simulink model "SF011A_EotLrng"  (R2013b)
settings: Solver=FixedStepDiscrete  SolverMode=SingleTasking  StartTime=0.0  StopTime=1  FixedStep=0.002  RelTol=1e-3
values from neighbouring files (symbols this model uses):
  ARCHGLBPRM_FLOATZEROTHD_ULS_F32 = DataDict.Constant    [SF011A_EotLrng_DataDict.m]
  CNVTOMILLISEC_MILLISECPERCNT_F32 = DataDict.Constant    [SF011A_EotLrng_DataDict.m]
  CORRLNFLT_CNT_U08 = DataDict.Constant    [SF011A_EotLrng_DataDict.m]
  DEBSTEP_CNT_U16 = DataDict.Constant    [SF011A_EotLrng_DataDict.m]
  EOTLIMDETD_CNT_LOGL = DataDict.Constant    [SF011A_EotLrng_DataDict.m]
  EOTLIMNOTDETD_CNT_LOGL = DataDict.Constant    [SF011A_EotLrng_DataDict.m]
  EotLrngAuthyStrtLrn = DataDict.Calibration    [SF011A_EotLrng_DataDict.m]
  EotLrngEotLrnTmr = DataDict.Calibration    [SF011A_EotLrng_DataDict.m]
  EotLrngHwAgOverTrvlCnt = DataDict.Calibration    [SF011A_EotLrng_DataDict.m]
  EotLrngHwAgOverTrvlEntr = DataDict.Calibration    [SF011A_EotLrng_DataDict.m]
  EotLrngHwAgOverTrvlExit = DataDict.Calibration    [SF011A_EotLrng_DataDict.m]
  EotLrngHwTqEotLrn = DataDict.Calibration    [SF011A_EotLrng_DataDict.m]
  EotLrngMotVelEotLrn = DataDict.Calibration    [SF011A_EotLrng_DataDict.m]
  EotLrngRackTrvlMax = DataDict.Calibration    [SF011A_EotLrng_DataDict.m]
  EotLrngRackTrvlMin = DataDict.Calibration    [SF011A_EotLrng_DataDict.m]
  EotLrngRstAuthyMin = DataDict.Calibration    [SF011A_EotLrng_DataDict.m]
  EotProtnRackTrvlLimrEna = DataDict.ImprtdCal    [SF011A_EotLrng_DataDict.m]
  HwAgOverTrvl = DataDict.NTC    [SF011A_EotLrng_DataDict.m]
  HWAGOVERTRVLMAXCNT_CNT_U08 = DataDict.Constant    [SF011A_EotLrng_DataDict.m]
  NODEBSTEP_CNT_U16 = DataDict.Constant    [SF011A_EotLrng_DataDict.m]
  OUTOFRNGFLT_CNT_U08 = DataDict.Constant    [SF011A_EotLrng_DataDict.m]
  RackEotStorgFlt = DataDict.NTC    [SF011A_EotLrng_DataDict.m]
  SIGAVLFLT_CNT_U08 = DataDict.Constant    [SF011A_EotLrng_DataDict.m]
undefined symbols (not defined in the file or in its folder): NtcSts1, NvmGetErrSts1, SigQlfr1
libraries: simulink x19, NxtrNvM x12, NxtrAbslt x5, NxtrLim x4, NxtrMax x3, NxtrMin x3
(part 7 of 7)

== system SF011A_EotLrng/EotLrng/EotLrngPer1/SRLNotEna/LrnEotLim/LrgnEotCmplSts/EotCwElpdTmr/GetTiSpan100MicroSec32bit/Wrapping/CopyRight2 ==

== stateflow chart SF011A_EotLrng/EotLrng/EotLrngPer1/SRLEna/ChkEotSigForNtc/EotSigAvl/SetCorrlFltNtc/SetNtcSts/ISO Fault Debounce Design ==
  note: NTCSTS_PASSD           (0)
      | NTCSTS_FAILD             (1)
      | NTCSTS_PREPASSD   (2)
      | NTCSTS_PREFAILD     (3)
      |
      | SIGQLFR_NORES        (0)
      | SIGQLFR_PASSD         (1)
      | SIGQLFR_FAILD           (2)
  note: Pass Loop
  note: Fail Loop
  note: 
  (default) -> (junction 89)
  (junction 89) -> (junction 95) [order 1] : [NtcSts ==3]
  (junction 89) -> (junction 93) [order 2] : [NtcSts ==2]
  (junction 89) -> (junction 141) [order 3] : [NtcSts ==1]
      | { ErrAcc = 32767;
      | Qualifier =2;
      |  }
  (junction 89) -> (junction 141) [order 4] : [NtcSts ==0]
      | { ErrAcc = -32768;
      | Qualifier=1;
      | }
  (junction 95) -> (junction 103) [order 2]
  (junction 95) -> (junction 111) [order 1] : [ErrAcc <=0]
      | {ErrAcc = DebStep;}
  (junction 93) -> (junction 123) [order 2] : {
      | ErrAcc = ErrAcc - DebStep;
      | }
  (junction 93) -> (junction 123) [order 1] : [(ErrAcc - DebStep) <= -32768]
      | { ErrAcc = -32768;
      | Qualifier=1;
      | }
  (junction 103) -> (junction 111) [order 1] : [(ErrAcc + DebStep) <32767]
      | {ErrAcc = ErrAcc + DebStep;}
  (junction 103) -> (junction 111) [order 2] : {ErrAcc = 32767;
      | Qualifier =2;}
  (junction 123) -> (junction 141)
  (junction 111) -> (junction 141)
  (junction 141) -> (junction 159) [order 2] : {ErrAcc = 0;
      | Qualifier =0;
      | }
  (junction 141) -> (junction 159) [order 1] : [SvcClr ==0]
  data: NtcSts input Enum: NtcSts1; Qualifier output uint8; DebStep input uint16; ErrAcc local single; SvcClr input

== stateflow chart SF011A_EotLrng/EotLrng/EotLrngPer1/SRLEna/ChkEotSigForNtc/SetSigAvlFltNtc/SetNtcSts/ISO Fault Debounce Design ==
  note: NTCSTS_PASSD           (0)
      | NTCSTS_FAILD             (1)
      | NTCSTS_PREPASSD   (2)
      | NTCSTS_PREFAILD     (3)
      |
      | SIGQLFR_NORES        (0)
      | SIGQLFR_PASSD         (1)
      | SIGQLFR_FAILD           (2)
  note: Pass Loop
  note: Fail Loop
  note: 
  (default) -> (junction 89)
  (junction 89) -> (junction 95) [order 1] : [NtcSts ==3]
  (junction 89) -> (junction 93) [order 2] : [NtcSts ==2]
  (junction 89) -> (junction 141) [order 3] : [NtcSts ==1]
      | { ErrAcc = 32767;
      | Qualifier =2;
      |  }
  (junction 89) -> (junction 141) [order 4] : [NtcSts ==0]
      | { ErrAcc = -32768;
      | Qualifier=1;
      | }
  (junction 95) -> (junction 103) [order 2]
  (junction 95) -> (junction 111) [order 1] : [ErrAcc <=0]
      | {ErrAcc = DebStep;}
  (junction 93) -> (junction 123) [order 2] : {
      | ErrAcc = ErrAcc - DebStep;
      | }
  (junction 93) -> (junction 123) [order 1] : [(ErrAcc - DebStep) <= -32768]
      | { ErrAcc = -32768;
      | Qualifier=1;
      | }
  (junction 103) -> (junction 111) [order 1] : [(ErrAcc + DebStep) <32767]
      | {ErrAcc = ErrAcc + DebStep;}
  (junction 103) -> (junction 111) [order 2] : {ErrAcc = 32767;
      | Qualifier =2;}
  (junction 123) -> (junction 141)
  (junction 111) -> (junction 141)
  (junction 141) -> (junction 159) [order 2] : {ErrAcc = 0;
      | Qualifier =0;
      | }
  (junction 141) -> (junction 159) [order 1] : [SvcClr ==0]
  data: NtcSts input Enum: NtcSts1; Qualifier output uint8; DebStep input uint16; ErrAcc local single; SvcClr input

== stateflow chart SF011A_EotLrng/EotLrng/EotLrngPer1/SRLEna/ChkEotSigForNtc/EotSigAvl/SetOutOfRngNtc/SetNtcSts/ISO Fault Debounce Design ==
  note: NTCSTS_PASSD           (0)
      | NTCSTS_FAILD             (1)
      | NTCSTS_PREPASSD   (2)
      | NTCSTS_PREFAILD     (3)
      |
      | SIGQLFR_NORES        (0)
      | SIGQLFR_PASSD         (1)
      | SIGQLFR_FAILD           (2)
  note: Pass Loop
  note: Fail Loop
  note: 
  (default) -> (junction 89)
  (junction 89) -> (junction 95) [order 1] : [NtcSts ==3]
  (junction 89) -> (junction 93) [order 2] : [NtcSts ==2]
  (junction 89) -> (junction 141) [order 3] : [NtcSts ==1]
      | { ErrAcc = 32767;
      | Qualifier =2;
      |  }
  (junction 89) -> (junction 141) [order 4] : [NtcSts ==0]
      | { ErrAcc = -32768;
      | Qualifier=1;
      | }
  (junction 95) -> (junction 103) [order 2]
  (junction 95) -> (junction 111) [order 1] : [ErrAcc <=0]
      | {ErrAcc = DebStep;}
  (junction 93) -> (junction 123) [order 2] : {
      | ErrAcc = ErrAcc - DebStep;
      | }
  (junction 93) -> (junction 123) [order 1] : [(ErrAcc - DebStep) <= -32768]
      | { ErrAcc = -32768;
      | Qualifier=1;
      | }
  (junction 103) -> (junction 111) [order 1] : [(ErrAcc + DebStep) <32767]
      | {ErrAcc = ErrAcc + DebStep;}
  (junction 103) -> (junction 111) [order 2] : {ErrAcc = 32767;
      | Qualifier =2;}
  (junction 123) -> (junction 141)
  (junction 111) -> (junction 141)
  (junction 141) -> (junction 159) [order 2] : {ErrAcc = 0;
      | Qualifier =0;
      | }
  (junction 141) -> (junction 159) [order 1] : [SvcClr ==0]
  data: NtcSts input Enum: NtcSts1; Qualifier output uint8; DebStep input uint16; ErrAcc local single; SvcClr input

== stateflow chart SF011A_EotLrng/EotLrng/EotLrngPer1/HwAgCwAndCcwMax/HwAgCwAndCcw/OverTrvlDiagc/CntOvrTrvlAndSetNTC/SetOverTrvlDiagc/SetNtcSts/ISO Fault Debounce Design ==
  note: NTCSTS_PASSD           (0)
      | NTCSTS_FAILD             (1)
      | NTCSTS_PREPASSD   (2)
      | NTCSTS_PREFAILD     (3)
      |
      | SIGQLFR_NORES        (0)
      | SIGQLFR_PASSD         (1)
      | SIGQLFR_FAILD           (2)
  note: Pass Loop
  note: Fail Loop
  note: 
  (default) -> (junction 89)
  (junction 89) -> (junction 95) [order 1] : [NtcSts ==3]
  (junction 89) -> (junction 93) [order 2] : [NtcSts ==2]
  (junction 89) -> (junction 141) [order 3] : [NtcSts ==1]
      | { ErrAcc = 32767;
      | Qualifier =2;
      |  }
  (junction 89) -> (junction 141) [order 4] : [NtcSts ==0]
      | { ErrAcc = -32768;
      | Qualifier=1;
      | }
  (junction 95) -> (junction 103) [order 2]
  (junction 95) -> (junction 111) [order 1] : [ErrAcc <=0]
      | {ErrAcc = DebStep;}
  (junction 93) -> (junction 123) [order 2] : {
      | ErrAcc = ErrAcc - DebStep;
      | }
  (junction 93) -> (junction 123) [order 1] : [(ErrAcc - DebStep) <= -32768]
      | { ErrAcc = -32768;
      | Qualifier=1;
      | }
  (junction 103) -> (junction 111) [order 1] : [(ErrAcc + DebStep) <32767]
      | {ErrAcc = ErrAcc + DebStep;}
  (junction 103) -> (junction 111) [order 2] : {ErrAcc = 32767;
      | Qualifier =2;}
  (junction 123) -> (junction 141)
  (junction 111) -> (junction 141)
  (junction 141) -> (junction 159) [order 2] : {ErrAcc = 0;
      | Qualifier =0;
      | }
  (junction 141) -> (junction 159) [order 1] : [SvcClr ==0]
  data: NtcSts input Enum: NtcSts1; Qualifier output uint8; DebStep input uint16; ErrAcc local single; SvcClr input

== stateflow chart SF011A_EotLrng/EotLrng/EotLrngInit1/SetOverTrvlDiagcPass/SetNtcSts/ISO Fault Debounce Design ==
  note: NTCSTS_PASSD           (0)
      | NTCSTS_FAILD             (1)
      | NTCSTS_PREPASSD   (2)
      | NTCSTS_PREFAILD     (3)
      |
      | SIGQLFR_NORES        (0)
      | SIGQLFR_PASSD         (1)
      | SIGQLFR_FAILD           (2)
  note: Pass Loop
  note: Fail Loop
  note: 
  (default) -> (junction 89)
  (junction 89) -> (junction 95) [order 1] : [NtcSts ==3]
  (junction 89) -> (junction 93) [order 2] : [NtcSts ==2]
  (junction 89) -> (junction 141) [order 3] : [NtcSts ==1]
      | { ErrAcc = 32767;
      | Qualifier =2;
      |  }
  (junction 89) -> (junction 141) [order 4] : [NtcSts ==0]
      | { ErrAcc = -32768;
      | Qualifier=1;
      | }
  (junction 95) -> (junction 103) [order 2]
  (junction 95) -> (junction 111) [order 1] : [ErrAcc <=0]
      | {ErrAcc = DebStep;}
  (junction 93) -> (junction 123) [order 2] : {
      | ErrAcc = ErrAcc - DebStep;
      | }
  (junction 93) -> (junction 123) [order 1] : [(ErrAcc - DebStep) <= -32768]
      | { ErrAcc = -32768;
      | Qualifier=1;
      | }
  (junction 103) -> (junction 111) [order 1] : [(ErrAcc + DebStep) <32767]
      | {ErrAcc = ErrAcc + DebStep;}
  (junction 103) -> (junction 111) [order 2] : {ErrAcc = 32767;
      | Qualifier =2;}
  (junction 123) -> (junction 141)
  (junction 111) -> (junction 141)
  (junction 141) -> (junction 159) [order 2] : {ErrAcc = 0;
      | Qualifier =0;
      | }
  (junction 141) -> (junction 159) [order 1] : [SvcClr ==0]
  data: NtcSts input Enum: NtcSts1; Qualifier output uint8; DebStep input uint16; ErrAcc local single; SvcClr input

== stateflow chart SF011A_EotLrng/EotLrng/EotLrngPer1/SRLEna/ChkEotSigForNtc/EotSigAvl/Update NVM/SetNTCPass/SetNtcSts/ISO Fault Debounce Design ==
  note: NTCSTS_PASSD           (0)
      | NTCSTS_FAILD             (1)
      | NTCSTS_PREPASSD   (2)
      | NTCSTS_PREFAILD     (3)
      |
      | SIGQLFR_NORES        (0)
      | SIGQLFR_PASSD         (1)
      | SIGQLFR_FAILD           (2)
  note: Pass Loop
  note: Fail Loop
  note: 
  (default) -> (junction 89)
  (junction 89) -> (junction 95) [order 1] : [NtcSts ==3]
  (junction 89) -> (junction 93) [order 2] : [NtcSts ==2]
  (junction 89) -> (junction 141) [order 3] : [NtcSts ==1]
      | { ErrAcc = 32767;
      | Qualifier =2;
      |  }
  (junction 89) -> (junction 141) [order 4] : [NtcSts ==0]
      | { ErrAcc = -32768;
      | Qualifier=1;
      | }
  (junction 95) -> (junction 103) [order 2]
  (junction 95) -> (junction 111) [order 1] : [ErrAcc <=0]
      | {ErrAcc = DebStep;}
  (junction 93) -> (junction 123) [order 2] : {
      | ErrAcc = ErrAcc - DebStep;
      | }
  (junction 93) -> (junction 123) [order 1] : [(ErrAcc - DebStep) <= -32768]
      | { ErrAcc = -32768;
      | Qualifier=1;
      | }
  (junction 103) -> (junction 111) [order 1] : [(ErrAcc + DebStep) <32767]
      | {ErrAcc = ErrAcc + DebStep;}
  (junction 103) -> (junction 111) [order 2] : {ErrAcc = 32767;
      | Qualifier =2;}
  (junction 123) -> (junction 141)
  (junction 111) -> (junction 141)
  (junction 141) -> (junction 159) [order 2] : {ErrAcc = 0;
      | Qualifier =0;
      | }
  (junction 141) -> (junction 159) [order 1] : [SvcClr ==0]
  data: NtcSts input Enum: NtcSts1; Qualifier output uint8; DebStep input uint16; ErrAcc local single; SvcClr input
